simulink model "W03_1_frame_check"  (R2024b)
settings: Solver=FixedStepDiscrete  StartTime=0.0  StopTime=0  FixedStep=Ts  RelTol=1e-3
values from neighbouring files (symbols this model uses):
  alt0 = 1.183941401541233    (= 1.18394140154)    [W03_setup.m]
  alt_s = 1.2479525180533528    (= 1.24795251805)    [W03_setup.m]
  lat0 = -33.72276870341191    (= -33.7227687034)    [W03_setup.m]
  lat_s = -33.72242651051122    (= -33.7224265105)    [W03_setup.m]
  lon0 = 150.67399057896623    (= 150.673990579)    [W03_setup.m]
  lon_s = 150.67398709806955    (= 150.673987098)    [W03_setup.m]
  qw_s = 0.8775317724700065    (= 0.87753177247)    [W03_setup.m]
  qx_s = -0.002985170390113125    (= -0.00298517039011)    [W03_setup.m]
  qy_s = 0.0052473626483582015    (= 0.00524736264836)    [W03_setup.m]
  qz_s = 0.4794804920417796    (= 0.479480492042)    [W03_setup.m]
  Ts = 0.05    [W03_setup.m]
settings Model: Creator=admin  LastModifiedBy=admin

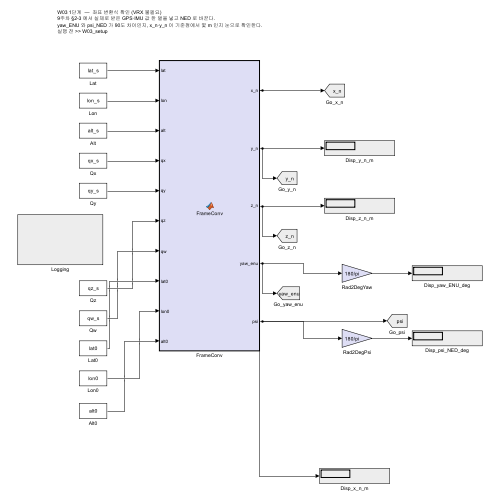
[thumbnail: Simulink's stored preview of the top-level diagram]
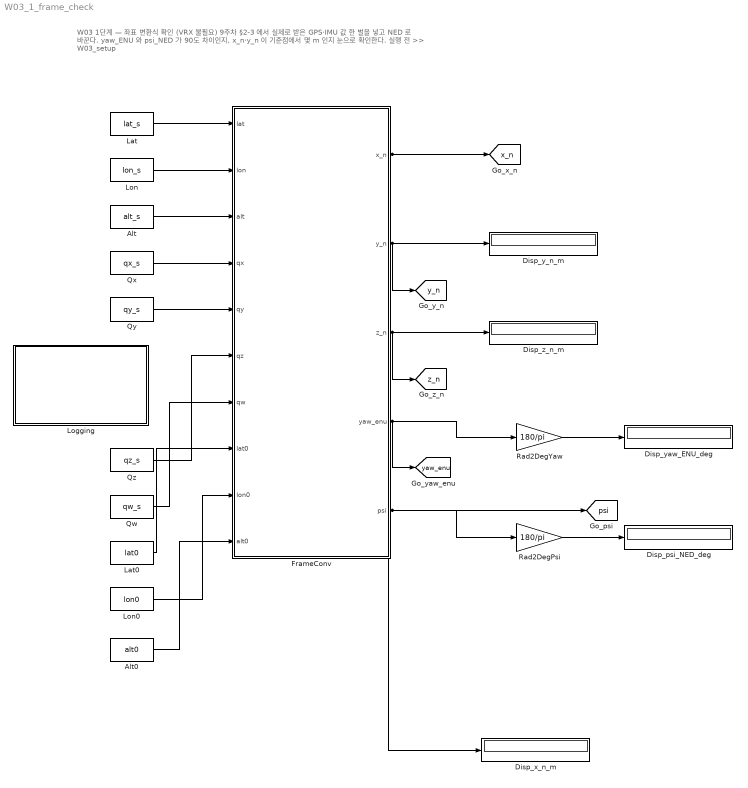
== system W03_1_frame_check ==
  note: W03 1단계  —  좌표 변환식 확인 (VRX 불필요)
      | 9주차 §2-3 에서 실제로 받은 GPS·IMU 값 한 벌을 넣고 NED 로 바꾼다.
      | yaw_ENU 와 psi_NED 가 90도 차이인지, x_n·y_n 이 기준점에서 몇 m 인지 눈으로 확인한다.
      | 실행 전 >> W03_setup
  Alt : Constant  Value=alt_s
  Alt0 : Constant  Value=alt0
  Disp_psi_NED_deg : Display
  Disp_x_n_m : Display
  Disp_y_n_m : Display
  Disp_yaw_ENU_deg : Display
  Disp_z_n_m : Display
  FrameConv : MATLAB Function  TreatAsAtomicUnit=on
  Lat : Constant  Value=lat_s
  Lat0 : Constant  Value=lat0
  Logging : Subsystem
  Lon : Constant  Value=lon_s
  Lon0 : Constant  Value=lon0
  Qw : Constant  Value=qw_s
  Qx : Constant  Value=qx_s
  Qy : Constant  Value=qy_s
  Qz : Constant  Value=qz_s
  Rad2DegPsi : Gain  Gain=180/pi
  Rad2DegYaw : Gain  Gain=180/pi
  tag scope: psi=global, x_n=global, y_n=global, yaw_enu=global, z_n=global
  wires:
  Lat/1 -> FrameConv/1(lat)
  Lon/1 -> FrameConv/2(lon)
  Alt/1 -> FrameConv/3(alt)
  Lat0/1 -> FrameConv/8(lat0)
  Qz/1 -> FrameConv/6(qz)
  Qx/1 -> FrameConv/4(qx)
  Qw/1 -> FrameConv/7(qw)
  Qy/1 -> FrameConv/5(qy)
  Lon0/1 -> FrameConv/9(lon0)
  Alt0/1 -> FrameConv/10(alt0)
  FrameConv/1(x_n) -> [x_n], Disp_x_n_m/1
  FrameConv/2(y_n) -> Disp_y_n_m/1, [y_n]
  FrameConv/3(z_n) -> Disp_z_n_m/1, [z_n]
  FrameConv/4(yaw_enu) -> Rad2DegYaw/1, [yaw_enu]
  FrameConv/5(psi) -> Rad2DegPsi/1, [psi]
  Rad2DegYaw/1 -> Disp_yaw_ENU_deg/1
  Rad2DegPsi/1 -> Disp_psi_NED_deg/1

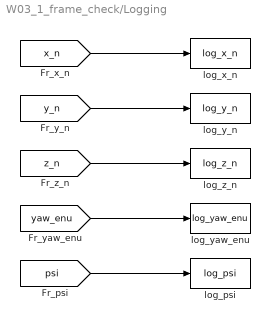
== system W03_1_frame_check/Logging ==
  log_psi : ToWorkspace  VariableName=log_psi  SaveFormat=Timeseries  SampleTime=Ts
  log_x_n : ToWorkspace  VariableName=log_x_n  SaveFormat=Timeseries  SampleTime=Ts
  log_y_n : ToWorkspace  VariableName=log_y_n  SaveFormat=Timeseries  SampleTime=Ts
  log_yaw_enu : ToWorkspace  VariableName=log_yaw_enu  SaveFormat=Timeseries  SampleTime=Ts
  log_z_n : ToWorkspace  VariableName=log_z_n  SaveFormat=Timeseries  SampleTime=Ts
  wires:
  [x_n] -> log_x_n/1
  [y_n] -> log_y_n/1
  [z_n] -> log_z_n/1
  [yaw_enu] -> log_yaw_enu/1
  [psi] -> log_psi/1

== matlab function W03_1_frame_check/FrameConv ==
  data: lat input; x_n output; lon input; alt input; qx input; qy input; qz input; qw input; lat0 input; lon0 input; alt0 input; y_n output; z_n output; yaw_enu output; psi output
function [x_n, y_n, z_n, yaw_enu, psi] = FrameConv(lat, lon, alt, qx, qy, qz, qw, lat0, lon0, alt0)
%#codegen
% ENU(ROS/Gazebo) -> NED(ship control). W03 section 1-5, 1-6.
%   position : flat-earth approximation around (lat0, lon0)
%   heading  : quaternion (ROS order x,y,z,w) -> yaw_ENU -> psi_NED

a  = 6378137.0;              % WGS84 semi-major axis [m]
e2 = 6.69437999014e-3;       % WGS84 first eccentricity squared

lat0r = lat0*pi/180;
s2    = sin(lat0r)^2;
Rm    = a*(1 - e2) / (1 - e2*s2)^1.5;      % meridian radius
Rn    = a / sqrt(1 - e2*s2);               % prime vertical radius

x_n =  (lat - lat0)*pi/180 * Rm;           % north [m]
y_n =  (lon - lon0)*pi/180 * Rn*cos(lat0r);% east  [m]
z_n = -(alt - alt0);                       % down  [m]

% yaw about ENU z (up). ROS quaternion order is (x, y, z, w).
yaw_enu = atan2(2*(qw*qz + qx*qy), 1 - 2*(qy*qy + qz*qz));
p   = pi/2 - yaw_enu;                      % NED heading
psi = atan2(sin(p), cos(p));               % wrap to [-pi, pi)
